simulink model "DP_PMP_MABX_2015a"  (R2015b)
settings: Solver=FixedStepDiscrete  StartTime=0.0  StopTime=60  FixedStep=60  RelTol=1e-3
PostLoadFcn:
  | , if any(exist('dsrtsu_mdlpostloadfcn', 'file') == [2, 3, 6]), try dsrtsu_mdlpostloadfcn('Execute', bdroot); catch fprintf('Error in PostLoadFcn (dsrtsu_mdlpostloadfcn) for model "%s":\n %s\n', bdroot, lasterr); end, end,
values from neighbouring files (symbols this model uses):
  FZG = par    [init.m]
undefined symbols (not defined in the file or in its folder): engKinMat_engKinInx_wayInx, engKinNum, engKinNumVec_wayInx, slpVec_wayInx, staNum, wayNum
settings Model: DSRTSU_INTERNAL_RTI_VER=440  DSRTSU_INTERNAL_RTI_TYPE=rti1401  DSRTSU_INTERNAL_RTIFPGA=30  Creator=Uebel  LastModifiedBy=kaulef
settings DataIOCC: SaveFormat=Array
settings DebuggingCC: ReadBeforeWriteMsg=DisableAll  WriteAfterWriteMsg=DisableAll  WriteAfterReadMsg=DisableAll  UnderspecifiedInitializationDetection=Classic  MergeDetectMultiDrivingBlocksExec=none  SolverPrmCheckMsg=warning  RootOutportRequireBusObject=error
settings HardwareCC: ProdBitPerPointer=32  ProdLargestAtomicFloat=None  ProdEndianess=BigEndian  ProdWordSize=32  ProdHWDeviceType=Generic->Custom  TargetIntDivRoundTo=Zero  TargetEndianess=BigEndian  TargetHWDeviceType=Generic->Custom
settings ModelReferenceCC: UpdateModelReferenceTargets=IfOutOfDate
settings SFSimCC: SFSimEcho=off
settings RTWCC: SystemTargetFile=rti1401.tlc  MakeCommand=make_rti  TemplateMakefile=rti1401.tmf  Description=dSPACE DS1401 Hardware Platform
settings STFCustomTargetCC: ParMdlRefBuildCompliant=on  ConcurrentExecutionCompliant=off  SystemTargetFile=rti1401.tlc
settings GRTTargetCC: CompOptLevelCompliant=off  ConcurrentExecutionCompliant=off  GeneratePreprocessorConditionals=Disable all  CombineOutputUpdateFcns=off  MatFileLogging=off  GRTInterface=on  UseToolchainInfoCompliant=off  ExtModeMexFile=noextcomm
settings ConfigComp: CovModelRefEnable=Off

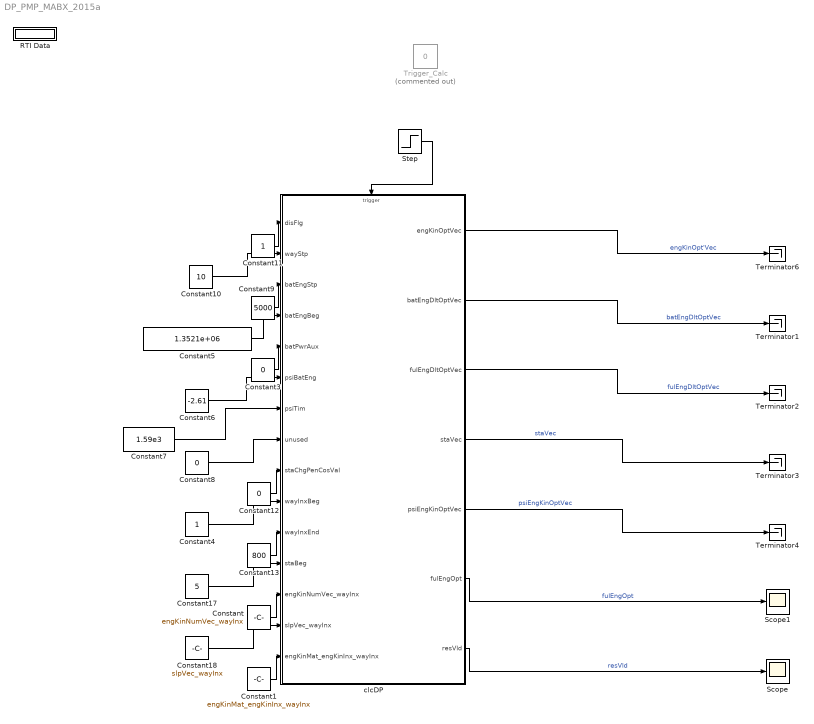
== system DP_PMP_MABX_2015a ==
  Constant : Constant  Value=engKinNumVec_wayInx
  Constant1 : Constant  Value=engKinMat_engKinInx_wayInx
  Constant10 : Constant  Value=10
  Constant11 : Constant
  Constant12 : Constant  Value=0
  Constant13 : Constant  Value=800
  Constant17 : Constant  Value=5
  Constant18 : Constant  Value=slpVec_wayInx
  Constant3 : Constant  Value=0
  Constant4 : Constant
  Constant5 : Constant  Value=1.3521e+06
  Constant6 : Constant  Value=-2.61
  Constant7 : Constant  Value=1.59e3
  Constant8 : Constant  Value=0
  Constant9 : Constant  Value=5000
  RTI Data : Subsystem  Tag=struct('RTIDataServer',struct('RTIDataServerVs','2','RTIModelDescription','struct(''main'',''DP_PMP_MABX_2013b'',''sub'','''',''isMp'',0)'))  LoadFcn="if exist('rtidc'), try,  rtidc('DataHostBlockClbLoad', gcbh); catch, disp(['Warning: ''LoadFcn'' for RTI Data block failed: ' lasterr]); end, end,"  mask(RTI_DATA_HOST){}
      mask help:
      | RTI Data Block.
      | This block is used by RTI to store internal model-dependent data.
      | Please keep this block on the root level of the model. Deleting this block will result in data loss.
      |
      | NEVER DELETE OR COPY THIS BLOCK!
      settings: CopyFcn="if exist('rtidc'), try,  rtidc('DataHostBlockClbCopy', gcbh); catch, disp(['Warning: ''CopyFcn'' for RTI Data block failed: ' lasterr]); end, end,"  DeleteFcn="if exist('rtidc'), try,  rtidc('DataHostBlockClbDelete', gcbh); catch, disp(['Warning: ''DeleteFcn'' for RTI Data block failed: ' lasterr]); end, end,"  ModelCloseFcn="if exist('rtidc'), try,  rtidc('DataHostBlockClbModelClose', gcbh); catch, disp(['Warning: ''ModelCloseFcn'' for RTI Data block failed: ' lasterr]); end, end,"  PreSaveFcn="if exist('rtidc'), try,  rtidc('DataHostBlockClbPreSave', gcbh); catch, disp(['Warning: ''PreSaveFcn'' for RTI Data block failed: ' lasterr]); end, end,"  PostSaveFcn="if exist('rtidc'), try,  rtidc('DataHostBlockClbPostSave', gcbh); catch, disp(['Warning: ''PostSaveFcn'' for RTI Data block failed: ' lasterr]); end, end,"  NameChangeFcn="if exist('rtidc'), try,  rtidc('DataHostBlockClbNameChange', gcbh); catch, disp(['Warning: ''NameChangeFcn'' for RTI Data block failed: ' lasterr]); end, end,"
      mask Help:
      | RTI Data Block.
      | This block is used by RTI to store internal model-dependent data.
      | Please keep this block on the root level of the model. Deleting this block will result in data loss.
      | 
      | NEVER DELETE OR COPY THIS BLOCK!
      mask Display:
      | text(0.5, 0.5, 'RTI Data', 'HorizontalAlignment', 'center');
      | plot([1 0]);
  Scope : Scope
  Scope1 : Scope
  Step : Step  SampleTime=0
  Terminator{1..4,6} (5 alike) : Terminator
  Trigger_Calc : Constant  Commented=on  Value=0
  clcDP : MATLAB Function  TreatAsAtomicUnit=on
  wires:
  Constant10/1 -> clcDP/2(wayStp)
  Constant11/1 -> clcDP/1(disFlg)
  Constant4/1 -> clcDP/10(wayInxBeg)
  Constant13/1 -> clcDP/11(wayInxEnd)
  Constant17/1 -> clcDP/12(staBeg)
  Constant/1 -> clcDP/13(engKinNumVec_wayInx)
  Constant1/1 -> clcDP/15(engKinMat_engKinInx_wayInx)
  Constant9/1 -> clcDP/3(batEngStp)
  Constant5/1 -> clcDP/4(batEngBeg)
  Constant3/1 -> clcDP/5(batPwrAux)
  Constant6/1 -> clcDP/6(psiBatEng)
  Constant7/1 -> clcDP/7(psiTim)
  Constant8/1 -> clcDP/8(unused)
  Constant12/1 -> clcDP/9(staChgPenCosVal)
  Constant18/1 -> clcDP/14(slpVec_wayInx)
  clcDP/1(engKinOptVec) -> Terminator6/1  "engKinOpt'Vec"
  clcDP/2(batEngDltOptVec) -> Terminator1/1  "batEngDltOptVec"
  clcDP/3(fulEngDltOptVec) -> Terminator2/1  "fulEngDltOptVec"
  clcDP/4(staVec) -> Terminator3/1  "staVec"
  clcDP/5(psiEngKinOptVec) -> Terminator4/1  "psiEngKinOptVec"
  clcDP/6(fulEngOpt) -> Scope1/1  "fulEngOpt"
  clcDP/7(resVld) -> Scope/1  "resVld"
  Step/1 -> clcDP/Trigger

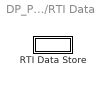
== system DP_PMP_MABX_2015a/RTI Data ==
  RTI Data Store : Subsystem  Tag="struct('private',struct('version',struct('dsVer',uint32(2),'dsVerCreation',uint32(2),'RTI',struct('ver','7.2','type','RTI1401')),'access',struct('type','Model','isPerm',1,'created',['29-Jan-2016 14:56:29'],'modified',['26-May-2016 10:11:47'],'location','')),'public',struct('main',struct('data',[]),'sub',struct('name',{{'DP_PMP_MABX_2013b'}},'data',{{struct('TH',struct('thTaskInfo',struct('taskType',{'TIMER','HWINT','TMRINT','SWINT','GLINT'},'tasksNumOf',{1,0,0,0,0},'srcIds',{{'TIMERA'},{},{},{},{}},'taskNames',{{['Timer Task 1']},{},{},{},{}})),'th_tc',struct('dataType','TASK','taskGroupId','','taskGroupList',{{}},'taskSchedulingPolicy','FCFS','taskType','TIMER','blkh',-1,'srcId','TIMERA','srcSgnName',['Timer A interrupt'],'srcCpuName','','taskName',['Timer Task 1  [60] s'],'taskNameDisplayExt','','smplTime',60,'smplTimeOffs',0,'hasFixedPriority',0,'priority',1,'hasFixedOvc',0,'ovcType',1,'ovcMax',1),'tc_th',struct('dataType','TASK','taskGroupId','','taskGroupList',{{}},'taskSchedulingPolicy','FCFS','taskType','TIMER','blkh',-1,'srcId','TIMERA','srcSgnName',['Timer A interrupt'],'srcCpuName','','taskName',['Timer Task 1  [60] s'],'taskNameDisplayExt','','smplTime',60,'smplTimeOffs',0,'hasFixedPriority',0,'priority',1,'hasFixedOvc',0,'ovcType',1,'ovcMax',1))}})))"  mask(RTI_DATA_STORE){}
      mask help:
      | RTI Data Store Block. This block is used by RTI to store internal model dependent data. Deleting this block will result in data loss.
      |
      | NEVER DELETE, COPY, OR MODIFY THIS BLOCK!
      mask Help:
      | RTI Data Store Block. This block is used by RTI to store internal model dependent data. Deleting this block will result in data loss.
      | 
      | NEVER DELETE, COPY, OR MODIFY THIS BLOCK!
      mask Display: text(0.5, 0.5, ' ', 'HorizontalAlignment', 'center');

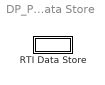
== system DP_PMP_MABX_2015a/RTI Data/RTI Data Store ==
  RTI Data Store : Subsystem  mask(RTI_DATA_STORE){}
      mask help:
      | RTI Data Store Block. This block is used by RTI to store internal model dependent data. Deleting this block will result in data loss.
      |
      | NEVER DELETE, COPY, OR MODIFY THIS BLOCK!
      mask Help:
      | RTI Data Store Block. This block is used by RTI to store internal model dependent data. Deleting this block will result in data loss.
      | 
      | NEVER DELETE, COPY, OR MODIFY THIS BLOCK!
      mask Display: text(0.5, 0.5, ' ', 'HorizontalAlignment', 'center');

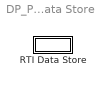
== system DP_PMP_MABX_2015a/RTI Data/RTI Data Store/RTI Data Store ==
  RTI Data Store : Subsystem  mask(RTI_DATA_STORE){}
      mask help:
      | RTI Data Store Block. This block is used by RTI to store internal model dependent data. Deleting this block will result in data loss.
      |
      | NEVER DELETE, COPY, OR MODIFY THIS BLOCK!
      mask Help:
      | RTI Data Store Block. This block is used by RTI to store internal model dependent data. Deleting this block will result in data loss.
      | 
      | NEVER DELETE, COPY, OR MODIFY THIS BLOCK!
      mask Display: text(0.5, 0.5, ' ', 'HorizontalAlignment', 'center');

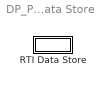
== system DP_PMP_MABX_2015a/RTI Data/RTI Data Store/RTI Data Store/RTI Data Store ==
  RTI Data Store : Subsystem  mask(RTI_DATA_STORE){}
      mask help:
      | RTI Data Store Block. This block is used by RTI to store internal model dependent data. Deleting this block will result in data loss.
      |
      | NEVER DELETE, COPY, OR MODIFY THIS BLOCK!
      mask Help:
      | RTI Data Store Block. This block is used by RTI to store internal model dependent data. Deleting this block will result in data loss.
      | 
      | NEVER DELETE, COPY, OR MODIFY THIS BLOCK!
      mask Display: text(0.5, 0.5, ' ', 'HorizontalAlignment', 'center');

== system DP_PMP_MABX_2015a/RTI Data/RTI Data Store/RTI Data Store/RTI Data Store/RTI Data Store ==

== matlab function DP_PMP_MABX_2015a/clcDP ==
  data: disFlg input; wayStp input; batEngStp input; batEngBeg input; batPwrAux input; psiBatEng input; psiTim input; unused input; staChgPenCosVal input; wayInxBeg input; wayInxEnd input; engKinNum parameter; staNum parameter; wayNum parameter; staBeg input; engKinNumVec_wayInx input; slpVec_wayInx input; engKinMat_engKinInx_wayInx input; engKinOptVec output; batEngDltOptVec output; fulEngDltOptVec output; staVec output; psiEngKinOptVec output; fulEngOpt output; resVld output; FZG parameter
  events: trigger_calculation input RISING_EDGE_EVENT
function ...            --- Ausgangsgrößen:
[engKinOptVec,...       Vektor - Trajektorie der optimalen kin. Energien
    batEngDltOptVec, ...Vektor - optimale Batterieenergieänderung
    fulEngDltOptVec,... Vektor - optimale Kraftstoffenergieänderung
    staVec,...          Vektor - Trajektorie des optimalen Antriebsstrangzustands
    psiEngKinOptVec,... Vektor - costate für kinetische Energie
    fulEngOpt, ...      Skalar - optimale Kraftstoffenergie
    resVld...
    ] = ...
    clcDP...
    ( ...               --- Eingangsgrößen:
    disFlg, ...         Skalar - Flag für Ausgabe in das Commandwindow
    wayStp,...          Skalar für die Wegschrittweite in m
    batEngStp,...       Skalar der Batteriediskretisierung in J
    batEngBeg,...       Skalar für die Batterieenergie am Beginn in Ws
    batPwrAux,...       Skalar für die Nebenverbrauchlast in W
    psiBatEng,...       Skalar für den Co-State der Batterieenergie
    psiTim,...          Skalar für den Co-State der Zeit
    ~, staChgPenCosVal,... Skalar für die Strafkosten beim Zustandswechsel
    wayInxBeg,...       Skalar für Anfangsindex in den Eingangsdaten
    wayInxEnd,...       Skalar für Endindex in den Eingangsdaten
    engKinNum,...       Skalar für die max. Anz. an engKin-Stützstellen
    staNum,...          Skalar für die max. Anzahl an Zustandsstützstellen
    wayNum,...          Skalar für die max. Anzahl an Wegstützstellen
    staBeg,...          Skalar für den Startzustand des Antriebsstrangs
    engKinNumVec_wayInx,... Vektor der Anzahl der kinetischen Energien
    slpVec_wayInx,...   Vektor der Steigungen in rad
    engKinMat_engKinInx_wayInx,... Matrix der kinetischen Energien in J%#codegen
    FZG)

%% Calculating optimal predecessors with DP + PMP
fprintf('Start\n');
[... --- Ausgangsgrößen:
    optPreInxTn3, ...   Tensor 3. Stufe für opt. Vorgängerkoordinaten
    batFrcOptTn3, ...   Tensor 3. Stufe der Batteriekraft
    fulEngOptTn3, ...   Tensor 3. Stufe für die Kraftstoffenergie 
    cos2goActMat ...    Matrix der optimalen Kosten der Hamiltonfunktion 
    ] = ... 
    clcDP_olyHyb...     FUNKTION
    ( ...               --- Eingangsgrößen:
    disFlg, ...         Skalar - Flag für Ausgabe in das Commandwindow
    wayStp,...          Skalar für die Wegschrittweite in m
    batEngStp,...       Skalar der Batteriediskretisierung in J
    batEngBeg,...       Skalar für die Batterieenergie am Beginn in Ws
    batPwrAux,...       Skalar für die Nebenverbrauchlast in W
    psiBatEng,...       Skalar für den Co-State der Batterieenergie
    psiTim,...          Skalar für den Co-State der Zeit
    [],...              Skalar für die Strafkosten für einen Motorstart
    staChgPenCosVal,... Skalar für die Strafkosten beim Zustandswechsel
    wayInxBeg,...       Skalar für Anfangsindex in den Eingangsdaten
    wayInxEnd,...       Skalar für Endindex in den Eingangsdaten
    1,...               Skalar für den Index der Anfangsgeschwindigkeit
    engKinNum,...       Skalar für die max. Anz. an engKin-Stützstellen
    staNum,...          Skalar für die max. Anzahl an Zustandsstützstellen
    wayNum,...          Skalar für die max. Anzahl an Wegstützstellen
    staBeg,...          Skalar für den Startzustand des Antriebsstrangs
    engKinNumVec_wayInx,... Vektor der Anzahl der kinetischen Energien
    slpVec_wayInx,...   Vektor der Steigungen in rad
    engKinMat_engKinInx_wayInx,... Matrix der kinetischen Energien in J
    FZG...              struct der Fahrzeugparameter
    );
engKinEndInxVal = ceil(engKinNumVec_wayInx(wayInxEnd)/2);
staEnd = staBeg;

%% Calculating optimal trajectories for result of DP + PMP
[engKinOptVec,...       Vektor - Trajektorie der optimalen kin. Energien
    batEngDltOptVec, ...Vektor - optimale Batterieenergieänderung
    fulEngDltOptVec,... Vektor - optimale Kraftstoffenergieänderung
    staVec,...          Vektor - Trajektorie des optimalen Antriebsstrangzustands
    psiEngKinOptVec,... Vektor - costate für kinetische Energie
    fulEngOpt ...       Skalar - optimale Kraftstoffenergie
    ] = ...
    clcOptTrj...        FUNKTION
    (false,...          Flag, ob Zielzustand genutzt werden muss
    wayStp,...          Skalar für die Wegschrittweite in m
    wayNum,...          Skalar für die max. Anzahl an Wegstützstellen
    wayInxBeg,...       Skalar für Anfangsindex in den Eingangsdaten
    wayInxEnd,...       Skalar für Endindex in den Eingangsdaten
    staEnd,...          Skalar für den finalen Zustand
    engKinNum,...       Skalar für die max. Anz. an engKin-Stützstellen
    engKinEndInxVal,... Skalar für Zielindex der kinetischen Energie
    staNum,...          Skalar für die max. Anzahl an Zustandsstützstellen
    engKinNumVec_wayInx,... Vektor der Anzahl der kinetischen Energien
    engKinMat_engKinInx_wayInx,... Matrix der kinetischen Energien in J
    optPreInxTn3,...    Tensor 3. Stufe für opt. Vorgängerkoordinaten
    batFrcOptTn3, ...   Tensor 3. Stufe der Batteriekraft
    fulEngOptTn3, ...   Tensor 3. Stufe für die Kraftstoffenergie
    cos2goActMat ...    Matrix der optimalen Kosten der Hamiltonfunktion 
    );

% engKinOptVec=0;
% batEngDltOptVec=0;
% fulEngDltOptVec=0;
% staVec=0;
% psiEngKinOptVec=0;
% fulEngOpt=0;
resVld = true;

fprintf('\n\nStop\n');
   
end
